simulink subsystem "parmeter_lookup_svsf"  (R2020b)
settings: Solver=VariableStepAuto  StartTime=0.0  StopTime=10.0  RelTol=1e-3
values from neighbouring files (symbols this model uses):
  delta = 0.1    [IMM_SVSF_VBL_init.m]
settings Model: Creator=Sara  LastModifiedBy=Sara

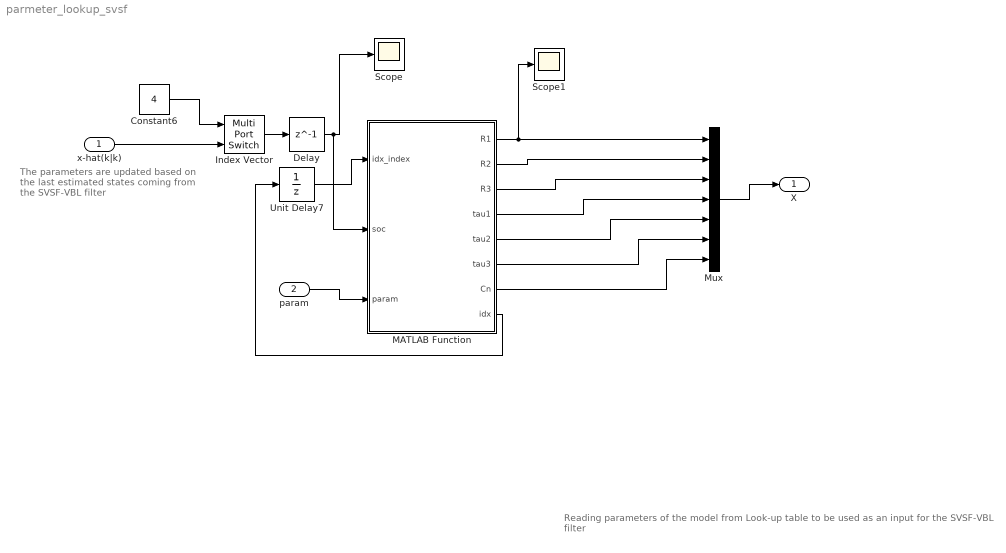
== system parmeter_lookup_svsf ==
  note: The parameters are updated based
      | on the last estimated states coming
      | from the SVSF-VBL filter
  note: Reading parameters of the model from Look-up table to be used as an input for the SVSF-VBL filter
  x-hat(k|k) : Inport
  param : Inport  Port=2
  Constant6 : Constant  Value=4  SampleTime=delta
  Delay : Delay  DelayLength=1  InitialCondition=.9
  Index Vector : MultiPortSwitch  Inputs=1
  MATLAB Function : MATLAB Function  TreatAsAtomicUnit=on
  Mux : Mux  Inputs=7
  Scope : Scope
  Scope1 : Scope
  Unit Delay7 : UnitDelay  SampleTime=-1  HasFrameUpgradeWarning=on
  X : Outport
  wires:
  param/1 -> MATLAB Function/3(param)
  x-hat(k|k)/1 -> Index Vector/2
  MATLAB Function/4(tau1) -> Mux/4
  MATLAB Function/3(R3) -> Mux/3
  Unit Delay7/1 -> MATLAB Function/1(idx_index)
  MATLAB Function/8(idx) -> Unit Delay7/1
  Constant6/1 -> Index Vector/1
  Index Vector/1 -> Delay/1
  MATLAB Function/7(Cn) -> Mux/7
  Mux/1 -> X/1
  MATLAB Function/6(tau3) -> Mux/6
  MATLAB Function/5(tau2) -> Mux/5
  MATLAB Function/2(R2) -> Mux/2
  MATLAB Function/1(R1) -> Mux/1, Scope1/1
  Delay/1 -> MATLAB Function/2(soc), Scope/1

== matlab function parmeter_lookup_svsf/MATLAB Function ==
  data: idx_index input; R1 output; soc input; param input; R2 output; R3 output; tau1 output; tau2 output; tau3 output; Cn output; idx output
function [R1, R2 , R3, tau1, tau2, tau3, Cn, idx] = GetModelParams( idx_index, soc, param)

    lkp_x = 0.2:.05:0.9;
    lkp_v = 1:15;
    % read the parameters based on the estimated SoC 
    idx =  interp1(lkp_x, lkp_v, soc , 'previous',15);
   
    R1 = param(1,idx);
    R2 = param(2,idx);
    R3 = param(3,idx);
    tau1 = param(4,idx);
    tau2 = param(5,idx);
    tau3 = param(6,idx);
    Cn = param(7,idx);
    
end
